simulink library "IOBlock_Library_TTC580"  (R2021a)
settings: Solver=ode45  StartTime=0.0  StopTime=10.0  RelTol=1e-3
PreLoadFcn:
  | addpath(genpath(fileparts(which('IOBlock_Library_TTC580'))));
  | %addpath(genpath(fileparts(which('IOBlock_Library_TTC580.mdl'))))
  | try
  | addpath(genpath([fileparts(which('IOBlock_Library_TTC580')),'\..\DBC_Importer']));
  | addpath(genpath([fileparts(which('IOBlock_Library_TTC580')),'\..\EEPROM_Importer']));
  | addpath(genpath([fileparts(which('IOBlock_Library_TTC580')),'\..\UserDoc']));
  | catch
  | warning('IOBlock_Library_TTC580: add path to DBC_Importer and EEPROM_Importer manually');
  | end
  | try
  | if exist('..\CustomPackage\scripts\OpenAllPackages.m','file')
  |      run('..\CustomPackage\scripts\OpenAllPackages.m'); %always available, ggf. empty
  | end
  | catch
  | warning('A problem occurred opening automatically the CustomPackage. Please open libraries manually');
  | end
  | try
  | set_param(0,'EditorSmartEditingHotParam','off');
  | catch
  | warning('Simlink preferences for ''Edit key parameter when adding new blocks'' needs to be unchecked manually');
  | end
undefined symbols (not defined in the file or in its folder): ADC_Absolute_10V, ADC_Absolute_32V, ADC_Absolute_5V, ADC_BoardTemp, ADC_ChannelInit, ADC_Current, ADC_Get, ADC_K15_, ADC_Ratiometric_10V, ADC_Ratiometric_5V, ADC_Resistive, ADC_SensorSupply, ADC_UBAT, bit_packing, bit_unpacking, CAN_ConfigMsg, compare2error, compare2FET_PROT_REENABLE, crc32_calc_intern, CRC32_EEPROM_Read, CRC32_EEPROM_Write, DIAG_EnterSafestate, DIAG_Status, DIAG_Status_internal, EEPROM_Mirror, EEPROM_Read, EEPROM_Read_OffsetIn, EEPROM_Read_Raw, EEPROM_Write, EEPROM_Write_OffsetIn, EEPROM_Write_Raw, EnterSafestate, FPU_Handler, Get_DI, Get_DI_VarThreshold, Get_K15_, Get_Pulse_Freq_Curr, Get_Pulse_Freq_Volt, Get_WakeUp, GetDateAndTime, IO_ADC_ResetProtection, IO_Blk_Lib_TTC500, IO_CAN_ReadMsg, IO_CAN_WriteMsg, IO_DI_Get, IO_DI_Init, IO_DI_Init_Var, IO_DO_GetCur, IO_DO_GetVoltage, IO_DO_Init, IO_DO_ResetProtection, IO_DO_Set, IO_Driver_GetSerialNumber, IO_Driver_GetVersionOfDriver, IO_Driver_GetVersionOfFPGA, IO_EEPROM_GetStatus, IO_EEPROM_Init, IO_EEPROM_Read_raw, IO_EEPROM_Write, IO_EEPROM_Write_OffsetIn ... (+73)
libraries: simulink x43
(part 13 of 18)

== system IOBlock_Library_TTC580/PWD Blocks TTC580 IOlib/Get_Pulse_Freq_Curr ==
  IO_PWD_ComplexGet : Subsystem  LoadFcn=|  mask(IO_PWD_ComplexGet_Code){SampleTime=-1, ttlib=IO_Blk_Lib_TTC500, ttDescription=IO_PWD_ComplexGet, tt_iolib_version=0.19, timer_channel=timer_channel, pin_value=NULL, pulse_samples=NULL}
      | try
      | %
      | %Upgrade Information - standard BEGIN
      | new_color = 'blue';
      | new_ver = '0.19';
      | act_ver = get_param(gcb,'tt_iolib_version');
      | if not(strcmp(act_ver,new_ver))
      |     disp(['Upgrade block: ',gcb,char(10),'       Version: ',act_ver,' -> ',new_ver]);
      |     %switch - case for specific upgrade information e.g. additional parameter required 
      |     %Change appearance and version information
      |     set_param(gcb,'ForegroundColor',new_color);
      |     set_param(gcb,'tt_iolib_version',new_ver);
      | end
      | %Upgrade Information - standard END
      | catch
      | %Standard catch section BEGIN 
      | disp(' ');
      | disp('------------------------------------------------------------');
      | disp('An error occurred in a callback of the TTC580-BlockLib.');
      | disp(['Please check the parameters in the mask of ',gcb]);
      | disp('If you do not encounter any violations, then please '); 
      | disp('copy the following lines and report this to support@ttcontrol.com ');
      | disp('<< begin of error message dump >>');
      | disp(['Version of TTC580-BlockLib: ', get_param(gcb,'tt_iolib_version')]);
      | disp(get_param(gcb,'ttDescription'));
      | disp(gcb);
      | x=lasterror;disp(x.message);
      | disp(get_param(gcb,'MaskValues'));
      | disp(version);
      | disp(computer);
      | disp('<< end of error message dump >>');
      | disp('------------------------------------------------------------');
      | disp(' ');
      | %Standard catch section END
      | end
      mask help: Get the frequency and the pulse-width from the specified timer channel.
      mask init:
      | %
      settings: CopyFcn=%deleted
      mask Help: No further help available for this block
      mask Callback timer_channel: %
      mask Callback pin_value: %
      mask Callback pulse_samples: %
  IO_PWD_ResetProtection : Subsystem  LoadFcn=|  mask(IO_PWD_ResetProtection_Code){SampleTime=-1, ttlib=IO_Blk_Lib_TTC500, ttDescription=IO_PWD_ResetProtection, tt_iolib_version=0.19, pwd_channel=timer_channel}
      | try
      | %
      | %Upgrade Information - standard BEGIN
      | new_color = 'blue';
      | new_ver = '0.19';
      | act_ver = get_param(gcb,'tt_iolib_version');
      | if not(strcmp(act_ver,new_ver))
      |     disp(['Upgrade block: ',gcb,char(10),'       Version: ',act_ver,' -> ',new_ver]);
      |     %switch - case for specific upgrade information e.g. additional parameter required 
      |     %Change appearance and version information
      |     set_param(gcb,'ForegroundColor',new_color);
      |     set_param(gcb,'tt_iolib_version',new_ver);
      | end
      | %Upgrade Information - standard END
      | catch
      | %Standard catch section BEGIN 
      | disp(' ');
      | disp('------------------------------------------------------------');
      | disp('An error occurred in a callback of the TTC580-BlockLib.');
      | disp(['Please check the parameters in the mask of ',gcb]);
      | disp('If you do not encounter any violations, then please '); 
      | disp('copy the following lines and report this to support@ttcontrol.com ');
      | disp('<< begin of error message dump >>');
      | disp(['Version of TTC580-BlockLib: ', get_param(gcb,'tt_iolib_version')]);
      | disp(get_param(gcb,'ttDescription'));
      | disp(gcb);
      | x=lasterror;disp(x.message);
      | disp(get_param(gcb,'MaskValues'));
      | disp(version);
      | disp(computer);
      | disp('<< end of error message dump >>');
      | disp('------------------------------------------------------------');
      | disp(' ');
      | %Standard catch section END
      | end
      mask help: Reset the FET protection for a timer input channel.
      mask init:
      | %
      settings: CopyFcn=%deleted
      mask Help: No further help available for this block
      mask Callback pwd_channel: %
  PWD_ComplexInit : Subsystem  LoadFcn=|  mask(PWD_ComplexInit_Code){SampleTime=-1, ttlib=IO_Blk_Lib_TTC500, ttDescription=PWD_ComplexInit, tt_iolib_version=0.19, timer_channel=timer_channel, pulse_mode=pulse_mode, freq_mode=freq_mode, capture_count=capture_count, pupd=pupd, safety_conf=NULL}
      | try
      | %
      | %Upgrade Information - standard BEGIN
      | new_color = 'blue';
      | new_ver = '0.19';
      | act_ver = get_param(gcb,'tt_iolib_version');
      | if not(strcmp(act_ver,new_ver))
      |     disp(['Upgrade block: ',gcb,char(10),'       Version: ',act_ver,' -> ',new_ver]);
      |     %switch - case for specific upgrade information e.g. additional parameter required 
      |     %Change appearance and version information
      |     set_param(gcb,'ForegroundColor',new_color);
      |     set_param(gcb,'tt_iolib_version',new_ver);
      | end
      | %Upgrade Information - standard END
      | catch
      | %Standard catch section BEGIN 
      | disp(' ');
      | disp('------------------------------------------------------------');
      | disp('An error occurred in a callback of the TTC580-BlockLib.');
      | disp(['Please check the parameters in the mask of ',gcb]);
      | disp('If you do not encounter any violations, then please '); 
      | disp('copy the following lines and report this to support@ttcontrol.com ');
      | disp('<< begin of error message dump >>');
      | disp(['Version of TTC580-BlockLib: ', get_param(gcb,'tt_iolib_version')]);
      | disp(get_param(gcb,'ttDescription'));
      | disp(gcb);
      | x=lasterror;disp(x.message);
      | disp(get_param(gcb,'MaskValues'));
      | disp(version);
      | disp(computer);
      | disp('<< end of error message dump >>');
      | disp('------------------------------------------------------------');
      | disp(' ');
      | %Standard catch section END
      | end
      mask help: Setup single timer channel that measures frequency and pulse-width at the same time.
      mask init:
      | %
      settings: CopyFcn=%deleted
      mask Help: No further help available for this block
      mask Callback timer_channel: %
      mask Callback pulse_mode: %
      mask Callback freq_mode: %
      mask Callback capture_count: %
      mask Callback pupd: %
      mask Callback safety_conf: %
  PWM_Init : Terminator
  Terminator1 : Terminator
  Terminator3 : Terminator
  compare2FET_PROT_REENABLE : Subsystem  LoadFcn=|  mask(compare2FET_PROT_REENABLE_Code){SampleTime=-1, ttlib=IO_Blk_Lib_TTC500, ttDescription=compare2FET_PROT_REENABLE, tt_iolib_version=0.19, define=IO_E_FET_PROT_REENABLE}
      | try
      | %
      | %Upgrade Information - standard BEGIN
      | new_color = 'blue';
      | new_ver = '0.19';
      | act_ver = get_param(gcb,'tt_iolib_version');
      | if not(strcmp(act_ver,new_ver))
      |     disp(['Upgrade block: ',gcb,char(10),'       Version: ',act_ver,' -> ',new_ver]);
      |     %switch - case for specific upgrade information e.g. additional parameter required 
      |     %Change appearance and version information
      |     set_param(gcb,'ForegroundColor',new_color);
      |     set_param(gcb,'tt_iolib_version',new_ver);
      | end
      | %Upgrade Information - standard END
      | catch
      | %Standard catch section BEGIN 
      | disp(' ');
      | disp('------------------------------------------------------------');
      | disp('An error occurred in a callback of the TTC580-BlockLib.');
      | disp(['Please check the parameters in the mask of ',gcb]);
      | disp('If you do not encounter any violations, then please '); 
      | disp('copy the following lines and report this to support@ttcontrol.com ');
      | disp('<< begin of error message dump >>');
      | disp(['Version of TTC580-BlockLib: ', get_param(gcb,'tt_iolib_version')]);
      | disp(get_param(gcb,'ttDescription'));
      | disp(gcb);
      | x=lasterror;disp(x.message);
      | disp(get_param(gcb,'MaskValues'));
      | disp(version);
      | disp(computer);
      | disp('<< end of error message dump >>');
      | disp('------------------------------------------------------------');
      | disp(' ');
      | %Standard catch section END
      | end
      mask help: The ErrorCode that is output from an I/O-Block is compared against IO_E_FET_PROT_REENABLE.
      mask init:
      | %
      settings: CopyFcn=%deleted
      mask Help: web(which('~.h'))
      mask Callback define: %
  ErrorCode : Outport  VectorParamsAs1DForOutWhenUnconnected=off
  frequency : Outport  Port=2  VectorParamsAs1DForOutWhenUnconnected=off
  pulse_width : Outport  Port=3  VectorParamsAs1DForOutWhenUnconnected=off
  wires:
  IO_PWD_ComplexGet/3(pulse_width) -> pulse_width/1
  IO_PWD_ComplexGet/2(frequency) -> frequency/1
  IO_PWD_ComplexGet/1(ErrorCode) -> ErrorCode/1, compare2FET_PROT_REENABLE/1(Errorcode)
  PWD_ComplexInit/1(ErrorCode) -> PWM_Init/1
  IO_PWD_ResetProtection/1(ErrorCode) -> Terminator3/1
  IO_PWD_ResetProtection/2(reset_cnt) -> Terminator1/1
  compare2FET_PROT_REENABLE/1(b_compare) -> IO_PWD_ResetProtection/Trigger

== system IOBlock_Library_TTC580/PWD Blocks TTC580 IOlib/Get_Pulse_Freq_Volt ==
  IO_PWD_ComplexGet : Subsystem  LoadFcn=|  mask(IO_PWD_ComplexGet_Code){SampleTime=-1, ttlib=IO_Blk_Lib_TTC500, ttDescription=IO_PWD_ComplexGet, tt_iolib_version=0.19, timer_channel=timer_channel, pin_value=NULL, pulse_samples=NULL}
      | try
      | %
      | %Upgrade Information - standard BEGIN
      | new_color = 'blue';
      | new_ver = '0.19';
      | act_ver = get_param(gcb,'tt_iolib_version');
      | if not(strcmp(act_ver,new_ver))
      |     disp(['Upgrade block: ',gcb,char(10),'       Version: ',act_ver,' -> ',new_ver]);
      |     %switch - case for specific upgrade information e.g. additional parameter required 
      |     %Change appearance and version information
      |     set_param(gcb,'ForegroundColor',new_color);
      |     set_param(gcb,'tt_iolib_version',new_ver);
      | end
      | %Upgrade Information - standard END
      | catch
      | %Standard catch section BEGIN 
      | disp(' ');
      | disp('------------------------------------------------------------');
      | disp('An error occurred in a callback of the TTC580-BlockLib.');
      | disp(['Please check the parameters in the mask of ',gcb]);
      | disp('If you do not encounter any violations, then please '); 
      | disp('copy the following lines and report this to support@ttcontrol.com ');
      | disp('<< begin of error message dump >>');
      | disp(['Version of TTC580-BlockLib: ', get_param(gcb,'tt_iolib_version')]);
      | disp(get_param(gcb,'ttDescription'));
      | disp(gcb);
      | x=lasterror;disp(x.message);
      | disp(get_param(gcb,'MaskValues'));
      | disp(version);
      | disp(computer);
      | disp('<< end of error message dump >>');
      | disp('------------------------------------------------------------');
      | disp(' ');
      | %Standard catch section END
      | end
      mask help: Get the frequency and the pulse-width from the specified timer channel.
      mask init:
      | %
      settings: CopyFcn=%deleted
      mask Help: No further help available for this block
      mask Callback timer_channel: %
      mask Callback pin_value: %
      mask Callback pulse_samples: %
  PWD_ComplexInit : Subsystem  LoadFcn=|  mask(PWD_ComplexInit_Code){SampleTime=-1, ttlib=IO_Blk_Lib_TTC500, ttDescription=PWD_ComplexInit, tt_iolib_version=0.19, timer_channel=timer_channel, pulse_mode=pulse_mode, freq_mode=freq_mode, capture_count=capture_count, pupd=pupd, safety_conf=NULL}
      | try
      | %
      | %Upgrade Information - standard BEGIN
      | new_color = 'blue';
      | new_ver = '0.19';
      | act_ver = get_param(gcb,'tt_iolib_version');
      | if not(strcmp(act_ver,new_ver))
      |     disp(['Upgrade block: ',gcb,char(10),'       Version: ',act_ver,' -> ',new_ver]);
      |     %switch - case for specific upgrade information e.g. additional parameter required 
      |     %Change appearance and version information
      |     set_param(gcb,'ForegroundColor',new_color);
      |     set_param(gcb,'tt_iolib_version',new_ver);
      | end
      | %Upgrade Information - standard END
      | catch
      | %Standard catch section BEGIN 
      | disp(' ');
      | disp('------------------------------------------------------------');
      | disp('An error occurred in a callback of the TTC580-BlockLib.');
      | disp(['Please check the parameters in the mask of ',gcb]);
      | disp('If you do not encounter any violations, then please '); 
      | disp('copy the following lines and report this to support@ttcontrol.com ');
      | disp('<< begin of error message dump >>');
      | disp(['Version of TTC580-BlockLib: ', get_param(gcb,'tt_iolib_version')]);
      | disp(get_param(gcb,'ttDescription'));
      | disp(gcb);
      | x=lasterror;disp(x.message);
      | disp(get_param(gcb,'MaskValues'));
      | disp(version);
      | disp(computer);
      | disp('<< end of error message dump >>');
      | disp('------------------------------------------------------------');
      | disp(' ');
      | %Standard catch section END
      | end
      mask help: Setup single timer channel that measures frequency and pulse-width at the same time.
      mask init:
      | %
      settings: CopyFcn=%deleted
      mask Help: No further help available for this block
      mask Callback timer_channel: %
      mask Callback pulse_mode: %
      mask Callback freq_mode: %
      mask Callback capture_count: %
      mask Callback pupd: %
      mask Callback safety_conf: %
  PWM_Init : Terminator
  ErrorCode : Outport  VectorParamsAs1DForOutWhenUnconnected=off
  frequency : Outport  Port=2  VectorParamsAs1DForOutWhenUnconnected=off
  pulse_width : Outport  Port=3  VectorParamsAs1DForOutWhenUnconnected=off
  wires:
  IO_PWD_ComplexGet/3(pulse_width) -> pulse_width/1
  IO_PWD_ComplexGet/2(frequency) -> frequency/1
  IO_PWD_ComplexGet/1(ErrorCode) -> ErrorCode/1
  PWD_ComplexInit/1(ErrorCode) -> PWM_Init/1

== system IOBlock_Library_TTC580/PWD Blocks TTC580 IOlib/PWD_Inc ==
  PWD_IncGet : Subsystem  LoadFcn=|  mask(PWD_IncGet_Code){SampleTime=-1, ttlib=IO_Blk_Lib_TTC500, ttDescription=PWD_IncGet, tt_iolib_version=0.19, inc_channel=inc_channel, pin_value_0=NULL, pin_value_1=NULL}
      | try
      | %
      | %Upgrade Information - standard BEGIN
      | new_color = 'blue';
      | new_ver = '0.19';
      | act_ver = get_param(gcb,'tt_iolib_version');
      | if not(strcmp(act_ver,new_ver))
      |     disp(['Upgrade block: ',gcb,char(10),'       Version: ',act_ver,' -> ',new_ver]);
      |     %switch - case for specific upgrade information e.g. additional parameter required 
      |     %Change appearance and version information
      |     set_param(gcb,'ForegroundColor',new_color);
      |     set_param(gcb,'tt_iolib_version',new_ver);
      | end
      | %Upgrade Information - standard END
      | catch
      | %Standard catch section BEGIN 
      | disp(' ');
      | disp('------------------------------------------------------------');
      | disp('An error occurred in a callback of the TTC580-BlockLib.');
      | disp(['Please check the parameters in the mask of ',gcb]);
      | disp('If you do not encounter any violations, then please '); 
      | disp('copy the following lines and report this to support@ttcontrol.com ');
      | disp('<< begin of error message dump >>');
      | disp(['Version of TTC580-BlockLib: ', get_param(gcb,'tt_iolib_version')]);
      | disp(get_param(gcb,'ttDescription'));
      | disp(gcb);
      | x=lasterror;disp(x.message);
      | disp(get_param(gcb,'MaskValues'));
      | disp(version);
      | disp(computer);
      | disp('<< end of error message dump >>');
      | disp('------------------------------------------------------------');
      | disp(' ');
      | %Standard catch section END
      | end
      mask help: Get the counter value of an incremental interface.
      mask init:
      | %
      settings: CopyFcn=%deleted
      mask Help: web(which('IO_PWD.h'))
      mask Callback inc_channel: %
      mask Callback pin_value_0: %
      mask Callback pin_value_1: %
  PWD_IncInit : Subsystem  LoadFcn=|  mask(PWD_IncInit_Code){SampleTime=-1, ttlib=IO_Blk_Lib_TTC500, ttDescription=PWD_IncInit, tt_iolib_version=0.19, inc_channel=inc_channel, mode=mode, count_init=num2str(0), pupd=pupd, safety_conf=NULL}
      | try
      | %
      | %Upgrade Information - standard BEGIN
      | new_color = 'blue';
      | new_ver = '0.19';
      | act_ver = get_param(gcb,'tt_iolib_version');
      | if not(strcmp(act_ver,new_ver))
      |     disp(['Upgrade block: ',gcb,char(10),'       Version: ',act_ver,' -> ',new_ver]);
      |     %switch - case for specific upgrade information e.g. additional parameter required 
      |     %Change appearance and version information
      |     set_param(gcb,'ForegroundColor',new_color);
      |     set_param(gcb,'tt_iolib_version',new_ver);
      | end
      | %Upgrade Information - standard END
      | catch
      | %Standard catch section BEGIN 
      | disp(' ');
      | disp('------------------------------------------------------------');
      | disp('An error occurred in a callback of the TTC580-BlockLib.');
      | disp(['Please check the parameters in the mask of ',gcb]);
      | disp('If you do not encounter any violations, then please '); 
      | disp('copy the following lines and report this to support@ttcontrol.com ');
      | disp('<< begin of error message dump >>');
      | disp(['Version of TTC580-BlockLib: ', get_param(gcb,'tt_iolib_version')]);
      | disp(get_param(gcb,'ttDescription'));
      | disp(gcb);
      | x=lasterror;disp(x.message);
      | disp(get_param(gcb,'MaskValues'));
      | disp(version);
      | disp(computer);
      | disp('<< end of error message dump >>');
      | disp('------------------------------------------------------------');
      | disp(' ');
      | %Standard catch section END
      | end
      mask help: Setup a single incremental interface.
      mask init:
      | %
      settings: CopyFcn=%deleted
      mask Help: web(which('IO_PWD.h'))
      mask Callback inc_channel: %
      mask Callback mode: %
      mask Callback count_init: %
      mask Callback pupd: %
      mask Callback safety_conf: %
  PWM_Init : Terminator
  ErrorCode : Outport  VectorParamsAs1DForOutWhenUnconnected=off
  count : Outport  Port=2  VectorParamsAs1DForOutWhenUnconnected=off
  wires:
  PWD_IncGet/1(ErrorCode) -> ErrorCode/1
  PWD_IncGet/2(count) -> count/1
  PWD_IncInit/1(ErrorCode) -> PWM_Init/1

== system IOBlock_Library_TTC580/PWD Blocks TTC580 IOlib/PWD_IncReset ==
  b_trigger : Inport  OutDataTypeStr=boolean  PortDimensions=1
  Constant : Constant  Value=count  OutDataTypeStr=uint16
  PWD_IncSet_Internal : Subsystem  LoadFcn=|  mask(PWD_IncSet_Internal_Code){SampleTime=-1, ttlib=IO_Blk_Lib_TTC500, ttDescription=PWD_IncSet_Internal, tt_iolib_version=0.19, inc_channel=inc_channel}
      | try
      | %
      | %Upgrade Information - standard BEGIN
      | new_color = 'blue';
      | new_ver = '0.19';
      | act_ver = get_param(gcb,'tt_iolib_version');
      | if not(strcmp(act_ver,new_ver))
      |     disp(['Upgrade block: ',gcb,char(10),'       Version: ',act_ver,' -> ',new_ver]);
      |     %switch - case for specific upgrade information e.g. additional parameter required 
      |     %Change appearance and version information
      |     set_param(gcb,'ForegroundColor',new_color);
      |     set_param(gcb,'tt_iolib_version',new_ver);
      | end
      | %Upgrade Information - standard END
      | catch
      | %Standard catch section BEGIN 
      | disp(' ');
      | disp('------------------------------------------------------------');
      | disp('An error occurred in a callback of the TTC580-BlockLib.');
      | disp(['Please check the parameters in the mask of ',gcb]);
      | disp('If you do not encounter any violations, then please '); 
      | disp('copy the following lines and report this to support@ttcontrol.com ');
      | disp('<< begin of error message dump >>');
      | disp(['Version of TTC580-BlockLib: ', get_param(gcb,'tt_iolib_version')]);
      | disp(get_param(gcb,'ttDescription'));
      | disp(gcb);
      | x=lasterror;disp(x.message);
      | disp(get_param(gcb,'MaskValues'));
      | disp(version);
      | disp(computer);
      | disp('<< end of error message dump >>');
      | disp('------------------------------------------------------------');
      | disp(' ');
      | %Standard catch section END
      | end
      mask help: Set the counter value of an incremental interface.
      mask init:
      | %
      settings: CopyFcn=%deleted
      mask Help: web(which('IO_PWD.h'))
      mask Callback inc_channel: %
  ErrorCode : Outport  VectorParamsAs1DForOutWhenUnconnected=off
  wires:
  PWD_IncSet_Internal/1(ErrorCode) -> ErrorCode/1
  Constant/1 -> PWD_IncSet_Internal/1(count)
  b_trigger/1 -> PWD_IncSet_Internal/Trigger

== system IOBlock_Library_TTC580/PWM Blocks TTC580 IOlib/Set_PWM_CurrFb ==
  duty_cycle : Inport  OutDataTypeStr=uint16  PortDimensions=1
  IO_PWM_GetCur : Subsystem  LoadFcn=|  mask(IO_PWM_GetCur_Code){SampleTime=-1, ttlib=IO_Blk_Lib_TTC500, ttDescription=IO_PWM_GetCur, tt_iolib_version=0.19, pwm_channel=pwm_channel}
      | try
      | %
      | %Upgrade Information - standard BEGIN
      | new_color = 'blue';
      | new_ver = '0.19';
      | act_ver = get_param(gcb,'tt_iolib_version');
      | if not(strcmp(act_ver,new_ver))
      |     disp(['Upgrade block: ',gcb,char(10),'       Version: ',act_ver,' -> ',new_ver]);
      |     %switch - case for specific upgrade information e.g. additional parameter required 
      |     %Change appearance and version information
      |     set_param(gcb,'ForegroundColor',new_color);
      |     set_param(gcb,'tt_iolib_version',new_ver);
      | end
      | %Upgrade Information - standard END
      | catch
      | %Standard catch section BEGIN 
      | disp(' ');
      | disp('------------------------------------------------------------');
      | disp('An error occurred in a callback of the TTC580-BlockLib.');
      | disp(['Please check the parameters in the mask of ',gcb]);
      | disp('If you do not encounter any violations, then please '); 
      | disp('copy the following lines and report this to support@ttcontrol.com ');
      | disp('<< begin of error message dump >>');
      | disp(['Version of TTC580-BlockLib: ', get_param(gcb,'tt_iolib_version')]);
      | disp(get_param(gcb,'ttDescription'));
      | disp(gcb);
      | x=lasterror;disp(x.message);
      | disp(get_param(gcb,'MaskValues'));
      | disp(version);
      | disp(computer);
      | disp('<< end of error message dump >>');
      | disp('------------------------------------------------------------');
      | disp(' ');
      | %Standard catch section END
      | end
      mask help: Returns the measured current of the given channel.
      mask init:
      | %
      settings: CopyFcn=%deleted
      mask Help: web(which('IO_PWM.h'))
      mask Callback pwm_channel: %
  IO_PWM_Init : Subsystem  LoadFcn=|  mask(IO_PWM_Init_Code){SampleTime=-1, ttlib=IO_Blk_Lib_TTC500, ttDescription=IO_PWM_Init, tt_iolib_version=0.19, pwm_channel=pwm_channel, frequency=frequency, polarity=num2str(polarity_high), diag_margin=num2str(diag_margin), safety_conf=NULL}
      | try
      | %
      | %Upgrade Information - standard BEGIN
      | new_color = 'blue';
      | new_ver = '0.19';
      | act_ver = get_param(gcb,'tt_iolib_version');
      | if not(strcmp(act_ver,new_ver))
      |     disp(['Upgrade block: ',gcb,char(10),'       Version: ',act_ver,' -> ',new_ver]);
      |     %switch - case for specific upgrade information e.g. additional parameter required 
      |     %Change appearance and version information
      |     set_param(gcb,'ForegroundColor',new_color);
      |     set_param(gcb,'tt_iolib_version',new_ver);
      | end
      | %Upgrade Information - standard END
      | catch
      | %Standard catch section BEGIN 
      | disp(' ');
      | disp('------------------------------------------------------------');
      | disp('An error occurred in a callback of the TTC580-BlockLib.');
      | disp(['Please check the parameters in the mask of ',gcb]);
      | disp('If you do not encounter any violations, then please '); 
      | disp('copy the following lines and report this to support@ttcontrol.com ');
      | disp('<< begin of error message dump >>');
      | disp(['Version of TTC580-BlockLib: ', get_param(gcb,'tt_iolib_version')]);
      | disp(get_param(gcb,'ttDescription'));
      | disp(gcb);
      | x=lasterror;disp(x.message);
      | disp(get_param(gcb,'MaskValues'));
      | disp(version);
      | disp(computer);
      | disp('<< end of error message dump >>');
      | disp('------------------------------------------------------------');
      | disp(' ');
      | %Standard catch section END
      | end
      mask help: Setup single PWM output.
      mask init:
      | %
      settings: CopyFcn=%deleted
      mask Help: web(which('IO_PWM.h'))
      mask Callback pwm_channel: %
      mask Callback frequency: %
      mask Callback polarity: %
      mask Callback diag_margin: %
      mask Callback safety_conf: %
  IO_PWM_ResetProtection : Subsystem  LoadFcn=|  mask(IO_PWM_ResetProtection_Code){SampleTime=-1, ttlib=IO_Blk_Lib_TTC500, ttDescription=IO_PWM_ResetProtection, tt_iolib_version=0.19, pwm_channel=pwm_channel}
      | try
      | %
      | %Upgrade Information - standard BEGIN
      | new_color = 'blue';
      | new_ver = '0.19';
      | act_ver = get_param(gcb,'tt_iolib_version');
      | if not(strcmp(act_ver,new_ver))
      |     disp(['Upgrade block: ',gcb,char(10),'       Version: ',act_ver,' -> ',new_ver]);
      |     %switch - case for specific upgrade information e.g. additional parameter required 
      |     %Change appearance and version information
      |     set_param(gcb,'ForegroundColor',new_color);
      |     set_param(gcb,'tt_iolib_version',new_ver);
      | end
      | %Upgrade Information - standard END
      | catch
      | %Standard catch section BEGIN 
      | disp(' ');
      | disp('------------------------------------------------------------');
      | disp('An error occurred in a callback of the TTC580-BlockLib.');
      | disp(['Please check the parameters in the mask of ',gcb]);
      | disp('If you do not encounter any violations, then please '); 
      | disp('copy the following lines and report this to support@ttcontrol.com ');
      | disp('<< begin of error message dump >>');
      | disp(['Version of TTC580-BlockLib: ', get_param(gcb,'tt_iolib_version')]);
      | disp(get_param(gcb,'ttDescription'));
      | disp(gcb);
      | x=lasterror;disp(x.message);
      | disp(get_param(gcb,'MaskValues'));
      | disp(version);
      | disp(computer);
      | disp('<< end of error message dump >>');
      | disp('------------------------------------------------------------');
      | disp(' ');
      | %Standard catch section END
      | end
      mask help: Reset the output protection for a PWM channel.
      mask init:
      | %
      settings: CopyFcn=%deleted
      mask Help: web(which('IO_PWM.h'))
      mask Callback pwm_channel: %
  PWM_Init : Terminator
  PWM_Init1 : Terminator
  PWM_Init2 : Terminator
  PWM_SetDuty_Simple : Subsystem  LoadFcn=|  mask(PWM_SetDuty_Simple_Code){SampleTime=-1, ttlib=IO_Blk_Lib_TTC500, ttDescription=PWM_SetDuty_Simple, tt_iolib_version=0.19, pwm_channel=pwm_channel, high_time_fb=NULL, period_fb=NULL}
      | try
      | %
      | %Upgrade Information - standard BEGIN
      | new_color = 'blue';
      | new_ver = '0.19';
      | act_ver = get_param(gcb,'tt_iolib_version');
      | if not(strcmp(act_ver,new_ver))
      |     disp(['Upgrade block: ',gcb,char(10),'       Version: ',act_ver,' -> ',new_ver]);
      |     %switch - case for specific upgrade information e.g. additional parameter required 
      |     %Change appearance and version information
      |     set_param(gcb,'ForegroundColor',new_color);
      |     set_param(gcb,'tt_iolib_version',new_ver);
      | end
      | %Upgrade Information - standard END
      | catch
      | %Standard catch section BEGIN 
      | disp(' ');
      | disp('------------------------------------------------------------');
      | disp('An error occurred in a callback of the TTC580-BlockLib.');
      | disp(['Please check the parameters in the mask of ',gcb]);
      | disp('If you do not encounter any violations, then please '); 
      | disp('copy the following lines and report this to support@ttcontrol.com ');
      | disp('<< begin of error message dump >>');
      | disp(['Version of TTC580-BlockLib: ', get_param(gcb,'tt_iolib_version')]);
      | disp(get_param(gcb,'ttDescription'));
      | disp(gcb);
      | x=lasterror;disp(x.message);
      | disp(get_param(gcb,'MaskValues'));
      | disp(version);
      | disp(computer);
      | disp('<< end of error message dump >>');
      | disp('------------------------------------------------------------');
      | disp(' ');
      | %Standard catch section END
      | end
      mask help: Set the duty cycle for a PWM channel.
      mask init:
      | %
      settings: CopyFcn=%deleted
      mask Help: web(which('IO_PWM.h'))
      mask Callback pwm_channel: %
      mask Callback high_time_fb: %
      mask Callback period_fb: %
  Terminator1 : Terminator
  Terminator3 : Terminator
  compare2FET_PROT_REENABLE : Subsystem  LoadFcn=|  mask(compare2FET_PROT_REENABLE_Code){SampleTime=-1, ttlib=IO_Blk_Lib_TTC500, ttDescription=compare2FET_PROT_REENABLE, tt_iolib_version=0.19, define=IO_E_FET_PROT_REENABLE}
      | try
      | %
      | %Upgrade Information - standard BEGIN
      | new_color = 'blue';
      | new_ver = '0.19';
      | act_ver = get_param(gcb,'tt_iolib_version');
      | if not(strcmp(act_ver,new_ver))
      |     disp(['Upgrade block: ',gcb,char(10),'       Version: ',act_ver,' -> ',new_ver]);
      |     %switch - case for specific upgrade information e.g. additional parameter required 
      |     %Change appearance and version information
      |     set_param(gcb,'ForegroundColor',new_color);
      |     set_param(gcb,'tt_iolib_version',new_ver);
      | end
      | %Upgrade Information - standard END
      | catch
      | %Standard catch section BEGIN 
      | disp(' ');
      | disp('------------------------------------------------------------');
      | disp('An error occurred in a callback of the TTC580-BlockLib.');
      | disp(['Please check the parameters in the mask of ',gcb]);
      | disp('If you do not encounter any violations, then please '); 
      | disp('copy the following lines and report this to support@ttcontrol.com ');
      | disp('<< begin of error message dump >>');
      | disp(['Version of TTC580-BlockLib: ', get_param(gcb,'tt_iolib_version')]);
      | disp(get_param(gcb,'ttDescription'));
      | disp(gcb);
      | x=lasterror;disp(x.message);
      | disp(get_param(gcb,'MaskValues'));
      | disp(version);
      | disp(computer);
      | disp('<< end of error message dump >>');
      | disp('------------------------------------------------------------');
      | disp(' ');
      | %Standard catch section END
      | end
      mask help: The ErrorCode that is output from an I/O-Block is compared against IO_E_FET_PROT_REENABLE.
      mask init:
      | %
      settings: CopyFcn=%deleted
      mask Help: web(which('~.h'))
      mask Callback define: %
  ErrorCode : Outport  VectorParamsAs1DForOutWhenUnconnected=off
  current : Outport  Port=2  VectorParamsAs1DForOutWhenUnconnected=off
  wires:
  IO_PWM_GetCur/2(current) -> current/1
  IO_PWM_Init/1(ErrorCode) -> PWM_Init/1
  duty_cycle/1 -> PWM_SetDuty_Simple/1(duty_cycle)
  PWM_SetDuty_Simple/1(ErrorCode) -> ErrorCode/1, compare2FET_PROT_REENABLE/1(Errorcode)
  IO_PWM_GetCur/1(ErrorCode) -> PWM_Init1/1
  IO_PWM_GetCur/3(fresh) -> PWM_Init2/1
  compare2FET_PROT_REENABLE/1(b_compare) -> IO_PWM_ResetProtection/Trigger
  IO_PWM_ResetProtection/1(ErrorCode) -> Terminator3/1
  IO_PWM_ResetProtection/2(reset_cnt) -> Terminator1/1

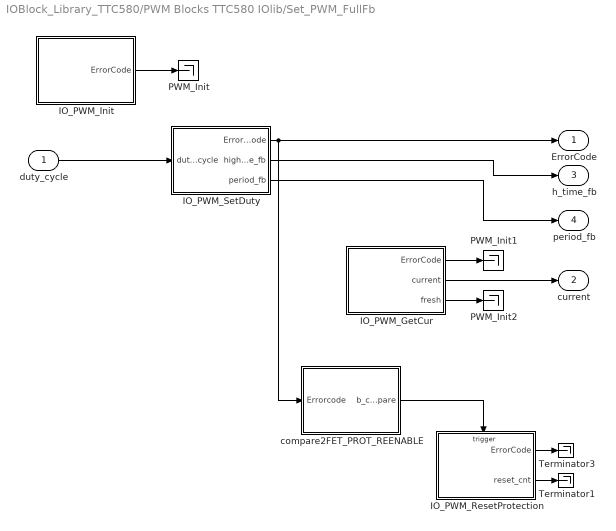
== system IOBlock_Library_TTC580/PWM Blocks TTC580 IOlib/Set_PWM_FullFb ==
  duty_cycle : Inport  OutDataTypeStr=uint16  PortDimensions=1
  IO_PWM_GetCur : Subsystem  LoadFcn=|  mask(IO_PWM_GetCur_Code){SampleTime=-1, ttlib=IO_Blk_Lib_TTC500, ttDescription=IO_PWM_GetCur, tt_iolib_version=0.19, pwm_channel=pwm_channel}
      | try
      | %
      | %Upgrade Information - standard BEGIN
      | new_color = 'blue';
      | new_ver = '0.19';
      | act_ver = get_param(gcb,'tt_iolib_version');
      | if not(strcmp(act_ver,new_ver))
      |     disp(['Upgrade block: ',gcb,char(10),'       Version: ',act_ver,' -> ',new_ver]);
      |     %switch - case for specific upgrade information e.g. additional parameter required 
      |     %Change appearance and version information
      |     set_param(gcb,'ForegroundColor',new_color);
      |     set_param(gcb,'tt_iolib_version',new_ver);
      | end
      | %Upgrade Information - standard END
      | catch
      | %Standard catch section BEGIN 
      | disp(' ');
      | disp('------------------------------------------------------------');
      | disp('An error occurred in a callback of the TTC580-BlockLib.');
      | disp(['Please check the parameters in the mask of ',gcb]);
      | disp('If you do not encounter any violations, then please '); 
      | disp('copy the following lines and report this to support@ttcontrol.com ');
      | disp('<< begin of error message dump >>');
      | disp(['Version of TTC580-BlockLib: ', get_param(gcb,'tt_iolib_version')]);
      | disp(get_param(gcb,'ttDescription'));
      | disp(gcb);
      | x=lasterror;disp(x.message);
      | disp(get_param(gcb,'MaskValues'));
      | disp(version);
      | disp(computer);
      | disp('<< end of error message dump >>');
      | disp('------------------------------------------------------------');
      | disp(' ');
      | %Standard catch section END
      | end
      mask help: Returns the measured current of the given channel.
      mask init:
      | %
      settings: CopyFcn=%deleted
      mask Help: web(which('IO_PWM.h'))
      mask Callback pwm_channel: %
  IO_PWM_Init : Subsystem  LoadFcn=|  mask(IO_PWM_Init_Code){SampleTime=-1, ttlib=IO_Blk_Lib_TTC500, ttDescription=IO_PWM_Init, tt_iolib_version=0.19, pwm_channel=pwm_channel, frequency=frequency, polarity=num2str(polarity_high), diag_margin=num2str(diag_margin), safety_conf=NULL}
      | try
      | %
      | %Upgrade Information - standard BEGIN
      | new_color = 'blue';
      | new_ver = '0.19';
      | act_ver = get_param(gcb,'tt_iolib_version');
      | if not(strcmp(act_ver,new_ver))
      |     disp(['Upgrade block: ',gcb,char(10),'       Version: ',act_ver,' -> ',new_ver]);
      |     %switch - case for specific upgrade information e.g. additional parameter required 
      |     %Change appearance and version information
      |     set_param(gcb,'ForegroundColor',new_color);
      |     set_param(gcb,'tt_iolib_version',new_ver);
      | end
      | %Upgrade Information - standard END
      | catch
      | %Standard catch section BEGIN 
      | disp(' ');
      | disp('------------------------------------------------------------');
      | disp('An error occurred in a callback of the TTC580-BlockLib.');
      | disp(['Please check the parameters in the mask of ',gcb]);
      | disp('If you do not encounter any violations, then please '); 
      | disp('copy the following lines and report this to support@ttcontrol.com ');
      | disp('<< begin of error message dump >>');
      | disp(['Version of TTC580-BlockLib: ', get_param(gcb,'tt_iolib_version')]);
      | disp(get_param(gcb,'ttDescription'));
      | disp(gcb);
      | x=lasterror;disp(x.message);
      | disp(get_param(gcb,'MaskValues'));
      | disp(version);
      | disp(computer);
      | disp('<< end of error message dump >>');
      | disp('------------------------------------------------------------');
      | disp(' ');
      | %Standard catch section END
      | end
      mask help: Setup single PWM output.
      mask init:
      | %
      settings: CopyFcn=%deleted
      mask Help: web(which('IO_PWM.h'))
      mask Callback pwm_channel: %
      mask Callback frequency: %
      mask Callback polarity: %
      mask Callback diag_margin: %
      mask Callback safety_conf: %
  IO_PWM_ResetProtection : Subsystem  LoadFcn=|  mask(IO_PWM_ResetProtection_Code){SampleTime=-1, ttlib=IO_Blk_Lib_TTC500, ttDescription=IO_PWM_ResetProtection, tt_iolib_version=0.19, pwm_channel=pwm_channel}
      | try
      | %
      | %Upgrade Information - standard BEGIN
      | new_color = 'blue';
      | new_ver = '0.19';
      | act_ver = get_param(gcb,'tt_iolib_version');
      | if not(strcmp(act_ver,new_ver))
      |     disp(['Upgrade block: ',gcb,char(10),'       Version: ',act_ver,' -> ',new_ver]);
      |     %switch - case for specific upgrade information e.g. additional parameter required 
      |     %Change appearance and version information
      |     set_param(gcb,'ForegroundColor',new_color);
      |     set_param(gcb,'tt_iolib_version',new_ver);
      | end
      | %Upgrade Information - standard END
      | catch
      | %Standard catch section BEGIN 
      | disp(' ');
      | disp('------------------------------------------------------------');
      | disp('An error occurred in a callback of the TTC580-BlockLib.');
      | disp(['Please check the parameters in the mask of ',gcb]);
      | disp('If you do not encounter any violations, then please '); 
      | disp('copy the following lines and report this to support@ttcontrol.com ');
      | disp('<< begin of error message dump >>');
      | disp(['Version of TTC580-BlockLib: ', get_param(gcb,'tt_iolib_version')]);
      | disp(get_param(gcb,'ttDescription'));
      | disp(gcb);
      | x=lasterror;disp(x.message);
      | disp(get_param(gcb,'MaskValues'));
      | disp(version);
      | disp(computer);
      | disp('<< end of error message dump >>');
      | disp('------------------------------------------------------------');
      | disp(' ');
      | %Standard catch section END
      | end
      mask help: Reset the output protection for a PWM channel.
      mask init:
      | %
      settings: CopyFcn=%deleted
      mask Help: web(which('IO_PWM.h'))
      mask Callback pwm_channel: %
  IO_PWM_SetDuty : Subsystem  LoadFcn=|  mask(IO_PWM_SetDuty_Code){SampleTime=-1, ttlib=IO_Blk_Lib_TTC500, ttDescription=IO_PWM_SetDuty, tt_iolib_version=0.19, pwm_channel=pwm_channel}
      | try
      | %
      | %Upgrade Information - standard BEGIN
      | new_color = 'blue';
      | new_ver = '0.19';
      | act_ver = get_param(gcb,'tt_iolib_version');
      | if not(strcmp(act_ver,new_ver))
      |     disp(['Upgrade block: ',gcb,char(10),'       Version: ',act_ver,' -> ',new_ver]);
      |     %switch - case for specific upgrade information e.g. additional parameter required 
      |     %Change appearance and version information
      |     set_param(gcb,'ForegroundColor',new_color);
      |     set_param(gcb,'tt_iolib_version',new_ver);
      | end
      | %Upgrade Information - standard END
      | catch
      | %Standard catch section BEGIN 
      | disp(' ');
      | disp('------------------------------------------------------------');
      | disp('An error occurred in a callback of the TTC580-BlockLib.');
      | disp(['Please check the parameters in the mask of ',gcb]);
      | disp('If you do not encounter any violations, then please '); 
      | disp('copy the following lines and report this to support@ttcontrol.com ');
      | disp('<< begin of error message dump >>');
      | disp(['Version of TTC580-BlockLib: ', get_param(gcb,'tt_iolib_version')]);
      | disp(get_param(gcb,'ttDescription'));
      | disp(gcb);
      | x=lasterror;disp(x.message);
      | disp(get_param(gcb,'MaskValues'));
      | disp(version);
      | disp(computer);
      | disp('<< end of error message dump >>');
      | disp('------------------------------------------------------------');
      | disp(' ');
      | %Standard catch section END
      | end
      mask help: Set the duty cycle for a PWM channel.
      mask init:
      | %
      settings: CopyFcn=%deleted
      mask Help: web(which('IO_PWM.h'))
      mask Callback pwm_channel: %
  PWM_Init : Terminator
  PWM_Init1 : Terminator
  PWM_Init2 : Terminator
  Terminator1 : Terminator
  Terminator3 : Terminator
  compare2FET_PROT_REENABLE : Subsystem  LoadFcn=|  mask(compare2FET_PROT_REENABLE_Code){SampleTime=-1, ttlib=IO_Blk_Lib_TTC500, ttDescription=compare2FET_PROT_REENABLE, tt_iolib_version=0.19, define=IO_E_FET_PROT_REENABLE}
      | try
      | %
      | %Upgrade Information - standard BEGIN
      | new_color = 'blue';
      | new_ver = '0.19';
      | act_ver = get_param(gcb,'tt_iolib_version');
      | if not(strcmp(act_ver,new_ver))
      |     disp(['Upgrade block: ',gcb,char(10),'       Version: ',act_ver,' -> ',new_ver]);
      |     %switch - case for specific upgrade information e.g. additional parameter required 
      |     %Change appearance and version information
      |     set_param(gcb,'ForegroundColor',new_color);
      |     set_param(gcb,'tt_iolib_version',new_ver);
      | end
      | %Upgrade Information - standard END
      | catch
      | %Standard catch section BEGIN 
      | disp(' ');
      | disp('------------------------------------------------------------');
      | disp('An error occurred in a callback of the TTC580-BlockLib.');
      | disp(['Please check the parameters in the mask of ',gcb]);
      | disp('If you do not encounter any violations, then please '); 
      | disp('copy the following lines and report this to support@ttcontrol.com ');
      | disp('<< begin of error message dump >>');
      | disp(['Version of TTC580-BlockLib: ', get_param(gcb,'tt_iolib_version')]);
      | disp(get_param(gcb,'ttDescription'));
      | disp(gcb);
      | x=lasterror;disp(x.message);
      | disp(get_param(gcb,'MaskValues'));
      | disp(version);
      | disp(computer);
      | disp('<< end of error message dump >>');
      | disp('------------------------------------------------------------');
      | disp(' ');
      | %Standard catch section END
      | end
      mask help: The ErrorCode that is output from an I/O-Block is compared against IO_E_FET_PROT_REENABLE.
      mask init:
      | %
      settings: CopyFcn=%deleted
      mask Help: web(which('~.h'))
      mask Callback define: %
  ErrorCode : Outport  VectorParamsAs1DForOutWhenUnconnected=off
  current : Outport  Port=2  VectorParamsAs1DForOutWhenUnconnected=off
  h_time_fb : Outport  Port=3  VectorParamsAs1DForOutWhenUnconnected=off
  period_fb : Outport  Port=4  VectorParamsAs1DForOutWhenUnconnected=off
  wires:
  IO_PWM_GetCur/2(current) -> current/1
  IO_PWM_Init/1(ErrorCode) -> PWM_Init/1
  duty_cycle/1 -> IO_PWM_SetDuty/1(duty_cycle)
  IO_PWM_SetDuty/1(ErrorCode) -> ErrorCode/1, compare2FET_PROT_REENABLE/1(Errorcode)
  IO_PWM_GetCur/1(ErrorCode) -> PWM_Init1/1
  IO_PWM_GetCur/3(fresh) -> PWM_Init2/1
  IO_PWM_SetDuty/2(high_time_fb) -> h_time_fb/1
  IO_PWM_SetDuty/3(period_fb) -> period_fb/1
  compare2FET_PROT_REENABLE/1(b_compare) -> IO_PWM_ResetProtection/Trigger
  IO_PWM_ResetProtection/1(ErrorCode) -> Terminator3/1
  IO_PWM_ResetProtection/2(reset_cnt) -> Terminator1/1
